simulink model "interfaceBasic"  (R2018b)
settings: Solver=FixedStepDiscrete  StartTime=0.0  StopTime=10.0  RelTol=1e-3
settings Model: Creator=matlab  LastModifiedBy=matlab
settings DataIOCC: SaveOutput=off  SignalLogging=off  SaveTime=off
settings OptimizationCC: DefaultParameterBehavior=Inlined  EnhancedBackFolding=on  PassReuseOutputArgsAs=Individual arguments  OptimizeBlockOrder=speed  DifferentSizesBufferReuse=on  OptimizationCustomize=off
settings DebuggingCC: ParameterTunabilityLossMsg=error
settings SFSimCC: MATLABDynamicMemAlloc=off
settings RTWCC: SystemTargetFile=ert.tlc  TemplateMakefile=ert_default_tmf  PostCodeGenCommand=packNGo(buildInfo);  GenerateReport=on  IncludeHyperlinkInReport=on  LaunchReport=on  GenerateTraceInfo=on  GenerateTraceReport=on  GenerateTraceReportSl=on  GenerateTraceReportSf=on  GenerateTraceReportEml=on
settings CodeAppCC: ForceParamTrailComments=on  IgnoreCustomStorageClasses=off  OperatorAnnotations=on  SimulinkDataObjDesc=on  SFDataObjDesc=on  InsertBlockDesc=on
settings ERTTargetCC: TargetLangStandard=C99 (ISO)  GenerateSampleERTMain=on  InlinedParameterPlacement=NonHierarchical  ERTCustomFileTemplate=example_file_process.tlc

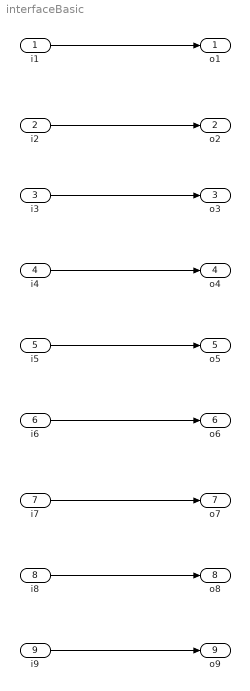
== system interfaceBasic ==
  i1 : Inport  OutDataTypeStr=MatLab_Double  BusOutputAsStruct=on
  i2 : Inport  Port=2  OutDataTypeStr=MatLab_Single  BusOutputAsStruct=on
  i3 : Inport  Port=3  OutDataTypeStr=MatLab_Int8  BusOutputAsStruct=on
  i4 : Inport  Port=4  OutDataTypeStr=MatLab_Uint8  BusOutputAsStruct=on
  i5 : Inport  Port=5  OutDataTypeStr=MatLab_Int16  BusOutputAsStruct=on
  i6 : Inport  Port=6  OutDataTypeStr=MatLab_Uint16  BusOutputAsStruct=on
  i7 : Inport  Port=7  OutDataTypeStr=MatLab_Int32  BusOutputAsStruct=on
  i8 : Inport  Port=8  OutDataTypeStr=MatLab_Uint32  BusOutputAsStruct=on
  i9 : Inport  Port=9  OutDataTypeStr=MatLab_Boolean  BusOutputAsStruct=on
  o1 : Outport  OutDataTypeStr=MatLab_Double
  o2 : Outport  Port=2  OutDataTypeStr=MatLab_Single
  o3 : Outport  Port=3  OutDataTypeStr=MatLab_Int8
  o4 : Outport  Port=4  OutDataTypeStr=MatLab_Uint8
  o5 : Outport  Port=5  OutDataTypeStr=MatLab_Int16
  o6 : Outport  Port=6  OutDataTypeStr=MatLab_Uint16
  o7 : Outport  Port=7  OutDataTypeStr=MatLab_Int32
  o8 : Outport  Port=8  OutDataTypeStr=MatLab_Uint32
  o9 : Outport  Port=9  OutDataTypeStr=MatLab_Boolean
  wires:
  i1/1 -> o1/1
  i2/1 -> o2/1
  i3/1 -> o3/1
  i4/1 -> o4/1
  i5/1 -> o5/1
  i6/1 -> o6/1
  i7/1 -> o7/1
  i8/1 -> o8/1
  i9/1 -> o9/1
